simulink library "wt_blockset_v3"  (Simulink 6.0)
settings: Solver=ode45  SolverMode=SingleTasking  StartTime=0.0  StopTime=10.0  RelTol=1e-3
undefined symbols (not defined in the file): f1, get, j, Kmode, Type, u0
libraries: simulink_extras x12, simulink3 x5, simulink x4, dspinverses x1, dspmtrx3 x1, dspsnks4 x1
(part 6 of 7)

== system wt_blockset_v3/Electrical Machinery/Simulink Blocks  based Models/RMS  Squirrel Cage Induction Machine/Steady State Model ==
  Vs : Inport  Port=1  LatchInput=off
  omg : Inport  Port=2  LatchInput=off
  Complex to Magnitude-Angle : ComplexToMagnitudeAngle
  Mux : Mux
  Mux1 : Mux  Inputs=2
  Product : Product  Inputs=*/  SaturateOnIntegerOverflow=on  InputSameDT=on
  Real-Imag to Complex : RealImagToComplex
  Selector : Selector  Elements=[1]  InputPortWidth=4
  electromagnetique torque : Fcn  Expr=3*p*Xm^2*u(1)^2*u(2)*u(3)/((Rs*u(3)+(Xm^2-Xs*u(4))*u(2))^2+(u(3)*Xs+u(2)*Rs*u(4))^2)/omg_base
  equivalent reactance : Fcn  Expr=(((u(3)/u(2))^2)*Xs-u(4)*(Xm^2-Xs*u(4)))/((u(3)/u(2))^2+u(4)^2)
  equivalent resistance : Fcn  Expr=(Rs*(u(3)/u(2))^2+Xm^2*u(3)/u(2)+Rs*u(4))/((u(3)/u(2))^2+u(4)^2)
  m<->g : Fcn  Expr=u(1)*(u(2) >=0)-(pi-u(1))*(u(2) < 0)
  rad->deg : Gain  Gain=180/pi  SaturateOnIntegerOverflow=on
  rotor reactance : Fcn  Expr=Xsgm_r*(abs(u(1))<=sbd)+(Xsgm_r*((kx-1)*abs(u(1))+(1-kx*sbd))/(1-sbd))*(abs(u(1))>sbd)+Xm
  rotor resistance : Fcn  Expr=Rr*(abs(u(1))<=sbd)+(Rr*((kr-1)*abs(u(1))+(1-kr*sbd))/(1-sbd))*(abs(u(1))>sbd)
  slip : Fcn  Expr=1-u(1)/omg_base
  Te : Outport
  Iph : Outport  Port=2
  phase_angle : Outport  Port=3
  wires:
  m<->g/1 -> rad->deg/1
  Mux1/1 -> m<->g/1
  Complex to Magnitude-Angle/2 -> Mux1/1
  Real-Imag to Complex/1 -> Complex to Magnitude-Angle/1
  Product/1 -> Iph/1
  Selector/1 -> Product/1
  Complex to Magnitude-Angle/1 -> Product/2
  rad->deg/1 -> phase_angle/1
  equivalent reactance/1 -> Real-Imag to Complex/2
  equivalent resistance/1 -> Real-Imag to Complex/1
  Mux/1 -> equivalent reactance/1, Selector/1, electromagnetique torque/1, equivalent resistance/1
  rotor reactance/1 -> Mux/4
  electromagnetique torque/1 -> Te/1
  rotor resistance/1 -> Mux/3
  slip/1 -> Mux1/2, rotor reactance/1, rotor resistance/1, Mux/2
  Vs/1 -> Mux/1
  omg/1 -> slip/1

== system wt_blockset_v3/Electrical Machinery/Simulink Blocks  based Models/Salient-Pole Synchronous Machine constant parameters/Mathematical model ==
  usdq : Inport  Port=1  LatchInput=off
  uf : Inport  Port=2  LatchInput=off
  omgr : Inport  Port=3  LatchInput=off
  Demux : Demux  Outputs=2
  Integrator{1..5} (5 alike) : Integrator
  Mux : Mux  Inputs=9
  Mux1 : Mux  Inputs=3
  Telm : Fcn  Expr=1.5*p*((Lmd-Lmq)*u[1]*u[2]+Lmq*u[2]*(u[3]+u[4])-Lmq*u[5]*u[1])
  dif/dt : Fcn  Expr=a31*u[1]+a32*u[9]*u[2]+a33*u[3]+a34*u[4]+a35*u[9]*u[5]+a36*u[6]+a37*u[8]
  dird/dt : Fcn  Expr=a41*u[1]+a42*u[9]*u[2]+a43*u[3]+a44*u[4]+a45*u[9]*u[5]+a46*u[6]+a47*u[8]
  dirq/dt : Fcn  Expr=a51*u[9]*u[1]+a52*u[2]+a53*u[9]*u[3]+a54*u[9]*u[4]+a55*u[5]+a56*u[7]
  disd/dt : Fcn  Expr=a11*u[1]+a12*u[9]*u[2]+a13*u[3]+a14*u[4]+a15*u[9]*u[5]+a16*u[6]+a17*u[8]
  disq/dt : Fcn  Expr=a21*u[9]*u[1]+a22*u[2]+a23*u[9]*u[3]+a24*u[9]*u[4]+a25*u[5]+a26*u[7]
  dq / abc : Subsystem
  isd : Selector  Elements=[1]  InputPortWidth=9
  isq : Selector  Elements=[2]  InputPortWidth=9
  Te : Outport  InitialOutput=0
  is_UVW : Outport  Port=2  InitialOutput=0
  wires:
  Mux/1 -> disd/dt/1, disq/dt/1, dif/dt/1, dird/dt/1, dirq/dt/1, Telm/1, isd/1, isq/1
  omgr/1 -> Mux/9
  uf/1 -> Mux/8
  disd/dt/1 -> Integrator4/1
  disq/dt/1 -> Integrator1/1
  dif/dt/1 -> Integrator2/1
  dird/dt/1 -> Integrator3/1
  dirq/dt/1 -> Integrator5/1
  Integrator5/1 -> Mux/5
  Integrator3/1 -> Mux/4
  Integrator2/1 -> Mux/3
  Integrator1/1 -> Mux/2
  Integrator4/1 -> Mux/1
  Telm/1 -> Te/1
  Demux/2 -> Mux/7
  Demux/1 -> Mux/6
  usdq/1 -> Demux/1
  dq / abc/1(A) -> Mux1/1
  dq / abc/2(B) -> Mux1/2
  dq / abc/3(C) -> Mux1/3
  Mux1/1 -> is_UVW/1
  [theta] -> dq / abc/3(theta)
  isd/1 -> dq / abc/1(D)
  isq/1 -> dq / abc/2(Q)

== system wt_blockset_v3/Electrical Machinery/Simulink Blocks  based Models/Salient-Pole Synchronous Machine constant parameters/abc-dq ==
  ABC : Inport  Port=1  LatchInput=off
  theta : Inport  Port=2  LatchInput=off
  Mux : Mux  Inputs=[3 1]
  Mux1 : Mux  Inputs=2
  d : Fcn  Expr=2*(u[1]*cos(u[4])+u[2]*cos(u[4]-2*pi/3)+u[3]*cos(u[4]+2*pi/3))/3
  q : Fcn  Expr=-2*(u[1]*sin(u[4])+u[2]*sin(u[4]-2*pi/3)+u[3]*sin(u[4]+2*pi/3))/3
  DQ : Outport  InitialOutput=0
  wires:
  Mux/1 -> d/1, q/1
  ABC/1 -> Mux/1
  Mux1/1 -> DQ/1
  d/1 -> Mux1/1
  q/1 -> Mux1/2
  theta/1 -> Mux/2

== system wt_blockset_v3/Electrical Machinery/Simulink Blocks  based Models/Squirrel Cage Induction Machine constant parameters/Derivatives ==
  vdqs : Inport  Port=1  LatchInput=off
  omega : Inport  Port=2  LatchInput=off
  Mux : Mux  Inputs=[1 1 1 1 2 1]
  Selector : Selector  Elements=[7]  InputPortWidth=7
  Selector1 : Selector  Elements=[1 2]  InputPortWidth=7
  didr/dt : Fcn  Expr=((Rs*Lm*u(1))/(Lss*Lsr)-Lm*u(7)*u(2)/Lsr-Rr*u(3)/Lsr-(Lm^2*u(7)*u(4))/(Lss*Lsr)-(Lm*u(5))/(Lss*Lsr))/sigma
  dids/dt : Fcn  Expr=(-Rs*u(1)/Lss+u(7)*u(2)+(Lm*Rr*u(3))/(Lss*Lsr)+Lm*u(7)*u(4)/Lss+u(5)/Lss)/sigma
  diqr/dt : Fcn  Expr=(Lm*u(7)*u(1)/Lsr+(Rs*Lm*u(2))/(Lss*Lsr)+(Lm^2*u(7)*u(3))/(Lss*Lsr)-Rr*u(4)/Lsr-(Lm*u(6))/(Lss*Lsr))/sigma
  diqs/dt : Fcn  Expr=(-u(7)*u(1)-Rs*u(2)/Lss-Lm*u(7)*u(3)/Lss+(Rr*Lm*u(4))/(Lss*Lsr)+u(6)/Lss)/sigma
  electromagnetique torque : Fcn  Expr=1.5*Lm*p*(u(2)*u(3)-u(1)*u(4))
  int_1 : Integrator  InitialCondition=x0(1)
  int_2 : Integrator  InitialCondition=x0(2)
  int_3 : Integrator  InitialCondition=x0(3)
  int_4 : Integrator  InitialCondition=x0(4)
  int_5 : Integrator  InitialCondition=x0(5)
  idqs : Outport
  Te : Outport  Port=2
  tag scope: theta=global
  wires:
  Selector1/1 -> idqs/1
  diqs/dt/1 -> int_2/1
  Selector/1 -> int_5/1
  int_5/1 -> [theta]  "theta"
  electromagnetique torque/1 -> Te/1
  diqr/dt/1 -> int_4/1
  didr/dt/1 -> int_3/1
  dids/dt/1 -> int_1/1
  Mux/1 -> Selector1/1, Selector/1, electromagnetique torque/1, diqr/dt/1, didr/dt/1, diqs/dt/1, dids/dt/1
  omega/1 -> Mux/6  "omega_rot"
  vdqs/1 -> Mux/5  "vdqs"
  int_4/1 -> Mux/4  "iqr"
  int_3/1 -> Mux/3  "idr"
  int_2/1 -> Mux/2  "iqs"
  int_1/1 -> Mux/1  "ids"

== system wt_blockset_v3/Electrical Machinery/Simulink Blocks  based Models/Squirrel Cage Induction Machine constant parameters/abc-dq ==
  ABC : Inport  Port=1  LatchInput=off
  theta : Inport  Port=2  LatchInput=off
  Mux : Mux  Inputs=[3 1]
  Mux1 : Mux  Inputs=2
  d : Fcn  Expr=2*(u[1]*cos(u[4])+u[2]*cos(u[4]-2*pi/3)+u[3]*cos(u[4]+2*pi/3))/3
  q : Fcn  Expr=-2*(u[1]*sin(u[4])+u[2]*sin(u[4]-2*pi/3)+u[3]*sin(u[4]+2*pi/3))/3
  DQ : Outport  InitialOutput=0
  wires:
  q/1 -> Mux1/2  "vqs"
  theta/1 -> Mux/2
  Mux1/1 -> DQ/1
  d/1 -> Mux1/1  "vds"
  ABC/1 -> Mux/1
  Mux/1 -> q/1, d/1

== system wt_blockset_v3/Electrical Machinery/Simulink Blocks  based Models/Squirrel Cage Induction Machine constant parameters/dq / abc ==
  DQ : Inport  Port=1  LatchInput=off
  theta : Inport  Port=2  LatchInput=off
  Mux : Mux  Inputs=[2 1]
  Mux1 : Mux  Inputs=3
  va : Fcn  Expr=u[1]*cos(u[3])-u[2]*sin(u[3])
  vb : Fcn  Expr=u[1]*cos(u[3]-2*pi/3)-u[2]*sin(u[3]-2*pi/3)
  vc : Fcn  Expr=u[1]*cos(u[3]+2*pi/3)-u[2]*sin(u[3]+2*pi/3)
  ABC : Outport  InitialOutput=0
  wires:
  theta/1 -> Mux/2
  Mux1/1 -> ABC/1
  vc/1 -> Mux1/3
  vb/1 -> Mux1/2
  va/1 -> Mux1/1
  DQ/1 -> Mux/1
  Mux/1 -> va/1, vb/1, vc/1

== system wt_blockset_v3/Electrical Machinery/Simulink Blocks  based Models/Squirrel Cage Induction Machine constant parameters/phase ->line ==
  In : Inport  Port=1  LatchInput=off
  Mux1 : Mux  Inputs=3
  iab : Fcn  Expr=u(1)-u(2)
  ibc : Fcn  Expr=u(2)-u(3)
  ica : Fcn  Expr=u(3)-u(1)
  Out : Outport
  wires:
  iab/1 -> Mux1/1
  ibc/1 -> Mux1/2
  ica/1 -> Mux1/3
  Mux1/1 -> Out/1
  In/1 -> iab/1, ibc/1, ica/1

== system wt_blockset_v3/Electrical Machinery/Simulink Blocks  based Models/Squirrel Cage  Induction Machine  with Deep Bar Effect/Derivatives ==
  note: DQ Model Of Squirrel-Cage Induction Machine with deep bar effect
  vdqs : Inport  Port=1  LatchInput=off
  omega : Inport  Port=2  LatchInput=off
  Mux : Mux  Inputs=[1 1 1 1 2 1 1 1]
  Selector : Selector  Elements=[7]  InputPortWidth=9
  Selector1 : Selector  Elements=[1 2]  InputPortWidth=9
  didr/dt : Fcn  Expr=((Rs*Lm*u(1))/(Lss*(u(9)+Lm))-Lm*u(7)*u(2)/(u(9)+Lm)-u(8)*u(3)/(u(9)+Lm)-(Lm^2*u(7)*u(4))/(Lss*(u(9)+Lm))-(Lm*u(5))/(Lss*(u(9)+Lm)))/(1-Lm^2/(Lss*(u(9)+Lm)))
  dids/dt : Fcn  Expr=(-Rs*u(1)/Lss+u(7)*u(2)+(Lm*u(8)*u(3))/(Lss*(u(9)+Lm))+Lm*u(7)*u(4)/Lss+u(5)/Lss)/(1-Lm^2/(Lss*(u(9)+Lm)))
  diqr/dt : Fcn  Expr=(Lm*u(7)*u(1)/(u(9)+Lm)+(Rs*Lm*u(2))/(Lss*(u(9)+Lm))+(Lm^2*u(7)*u(3))/(Lss*(u(9)+Lm))-u(8)*u(4)/(u(9)+Lm)-(Lm*u(6))/(Lss*(u(9)+Lm)))/(1-Lm^2/(Lss*(u(9)+Lm)))
  diqs/dt : Fcn  Expr=(-u(7)*u(1)-Rs*u(2)/Lss-Lm*u(7)*u(3)/Lss+(u(8)*Lm*u(4))/(Lss*(u(9)+Lm))+u(6)/Lss)/(1-Lm^2/(Lss*(u(9)+Lm)))
  electromagnetic torque : Fcn  Expr=1.5*Lm*p*(u(2)*u(3)-u(1)*u(4))
  int_1 : Integrator  InitialCondition=x0(1)
  int_2 : Integrator  InitialCondition=x0(2)
  int_3 : Integrator  InitialCondition=x0(3)
  int_4 : Integrator  InitialCondition=x0(4)
  int_5 : Integrator  InitialCondition=x0(5)
  rotor reactance : Fcn  Expr=Lsgmr*(abs(u(1))<=sbd)+(Lsgmr*((kx-1)*abs(u(1))+(1-kx*sbd))/(1-sbd))*(abs(u(1))>sbd)
  rotor resistance : Fcn  Expr=Rr*(abs(u(1))<=sbd)+(Rr*((kr-1)*abs(u(1))+(1-kr*sbd))/(1-sbd))*(abs(u(1))>sbd)
  slip : Fcn  Expr=1-u(1)/omg_base
  idqs : Outport
  Te : Outport  Port=2
  tag scope: theta=global
  wires:
  rotor reactance/1 -> Mux/8
  slip/1 -> rotor reactance/1, rotor resistance/1  "omega_rot"
  rotor resistance/1 -> Mux/7
  Selector1/1 -> idqs/1
  diqs/dt/1 -> int_2/1
  Selector/1 -> int_5/1
  int_5/1 -> [theta]  "theta"
  electromagnetic torque/1 -> Te/1
  diqr/dt/1 -> int_4/1
  didr/dt/1 -> int_3/1
  dids/dt/1 -> int_1/1
  Mux/1 -> Selector1/1, Selector/1, electromagnetic torque/1, diqr/dt/1, didr/dt/1, diqs/dt/1, dids/dt/1
  omega/1 -> Mux/6, slip/1  "omega_rot"
  vdqs/1 -> Mux/5  "vdqs"
  int_4/1 -> Mux/4  "iqr"
  int_3/1 -> Mux/3  "idr"
  int_2/1 -> Mux/2  "iqs"
  int_1/1 -> Mux/1  "ids"

== system wt_blockset_v3/Electrical Machinery/Simulink Blocks  based Models/Squirrel Cage  Induction Machine  with Deep Bar Effect/Subsystem1 ==
  DQ : Inport  Port=1  LatchInput=off
  theta : Inport  Port=2  LatchInput=off
  Mux : Mux  Inputs=[2 1]
  Mux1 : Mux  Inputs=3
  va : Fcn  Expr=u[1]*cos(u[3])-u[2]*sin(u[3])
  vb : Fcn  Expr=u[1]*cos(u[3]-2*pi/3)-u[2]*sin(u[3]-2*pi/3)
  vc : Fcn  Expr=u[1]*cos(u[3]+2*pi/3)-u[2]*sin(u[3]+2*pi/3)
  ABC : Outport  InitialOutput=0
  wires:
  theta/1 -> Mux/2
  Mux1/1 -> ABC/1
  vc/1 -> Mux1/3
  vb/1 -> Mux1/2
  va/1 -> Mux1/1
  DQ/1 -> Mux/1
  Mux/1 -> va/1, vb/1, vc/1

== system wt_blockset_v3/Electrical Machinery/Simulink Blocks  based Models/Squirrel Cage  Induction Machine  with Deep Bar Effect/abc-dq ==
  ABC : Inport  Port=1  LatchInput=off
  theta : Inport  Port=2  LatchInput=off
  Mux : Mux  Inputs=[3 1]
  Mux1 : Mux  Inputs=2
  d : Fcn  Expr=2*(u[1]*cos(u[4])+u[2]*cos(u[4]-2*pi/3)+u[3]*cos(u[4]+2*pi/3))/3
  q : Fcn  Expr=-2*(u[1]*sin(u[4])+u[2]*sin(u[4]-2*pi/3)+u[3]*sin(u[4]+2*pi/3))/3
  DQ : Outport  InitialOutput=0
  wires:
  q/1 -> Mux1/2  "vqs"
  theta/1 -> Mux/2
  Mux1/1 -> DQ/1
  d/1 -> Mux1/1  "vds"
  ABC/1 -> Mux/1
  Mux/1 -> q/1, d/1

== system wt_blockset_v3/Electrical Machinery/Simulink Blocks  based Models/Squirrel Cage  Induction Machine  with Deep Bar Effect/phase ->line ==
  In : Inport  Port=1  LatchInput=off
  Mux1 : Mux  Inputs=3
  iab : Fcn  Expr=u(1)-u(2)
  ibc : Fcn  Expr=u(2)-u(3)
  ica : Fcn  Expr=u(3)-u(1)
  Out : Outport
  wires:
  In/1 -> ica/1, ibc/1, iab/1
  Mux1/1 -> Out/1
  ica/1 -> Mux1/3
  ibc/1 -> Mux1/2
  iab/1 -> Mux1/1

== system wt_blockset_v3/Electrical Machinery/Simulink Blocks  based Models/Wound Rotor Induction Machine constant parameters/Subsystem1 ==
  DQ : Inport  Port=1  LatchInput=off
  theta : Inport  Port=2  LatchInput=off
  Mux : Mux  Inputs=[2 1]
  Mux1 : Mux  Inputs=3
  va : Fcn  Expr=u[1]*cos(u[3])-u[2]*sin(u[3])
  vb : Fcn  Expr=u[1]*cos(u[3]-2*pi/3)-u[2]*sin(u[3]-2*pi/3)
  vc : Fcn  Expr=u[1]*cos(u[3]+2*pi/3)-u[2]*sin(u[3]+2*pi/3)
  ABC : Outport  InitialOutput=0
  wires:
  theta/1 -> Mux/2
  Mux1/1 -> ABC/1
  vc/1 -> Mux1/3
  vb/1 -> Mux1/2
  va/1 -> Mux1/1
  DQ/1 -> Mux/1
  Mux/1 -> va/1, vb/1, vc/1

== system wt_blockset_v3/Electrical Machinery/Simulink Blocks  based Models/Wound Rotor Induction Machine constant parameters/Subsystem2 ==
  DQ : Inport  Port=1  LatchInput=off
  theta : Inport  Port=2  LatchInput=off
  Mux : Mux  Inputs=[2 1]
  Mux1 : Mux  Inputs=3
  va : Fcn  Expr=u[1]*cos(u[3])-u[2]*sin(u[3])
  vb : Fcn  Expr=u[1]*cos(u[3]-2*pi/3)-u[2]*sin(u[3]-2*pi/3)
  vc : Fcn  Expr=u[1]*cos(u[3]+2*pi/3)-u[2]*sin(u[3]+2*pi/3)
  ABC : Outport  InitialOutput=0
  wires:
  theta/1 -> Mux/2
  Mux/1 -> vc/1, vb/1, va/1
  DQ/1 -> Mux/1
  va/1 -> Mux1/1
  vb/1 -> Mux1/2
  vc/1 -> Mux1/3
  Mux1/1 -> ABC/1

== system wt_blockset_v3/Electrical Machinery/Simulink Blocks  based Models/Wound Rotor Induction Machine constant parameters/Voltage equations ==
  vdqs : Inport  Port=1  LatchInput=off
  vdqr : Inport  Port=2  LatchInput=off
  omega : Inport  Port=3  LatchInput=off
  Mux : Mux  Inputs=[1 1 1 1 2 2 1]
  Selector : Selector  Elements=[1 2]  InputPortWidth=9
  Selector1 : Selector  Elements=[3 4]  InputPortWidth=9
  Selector2 : Selector  Elements=[9]  InputPortWidth=9
  didr/dt : Fcn  Expr=(Rs*Lm*u(1)/(Lss*Lsr)-Lm*u(9)*u(2)/Lsr-Rr*u(3)/Lsr-((Lm^2)*u(9)*u(4))/(Lss*Lsr)-Lm*u(5)/(Lss*Lsr)+u(7)/Lsr)/sigma
  dids/dt : Fcn  Expr=(-Rs*u(1)/Lss+u(9)*u(2)+(Lm*Rr*u(3))/(Lss*Lsr)+Lm*u(9)*u(4)/Lss+u(5)/Lss-Lm*u(7)/(Lss*Lsr))/sigma
  diqr/dt : Fcn  Expr=(Lm*u(9)*u(1)/Lsr+Rs*Lm*u(2)/(Lss*Lsr)+((Lm^2)*u(9)*u(3))/(Lss*Lsr)-Rr*u(4)/Lsr-Lm*u(6)/(Lss*Lsr)+u(8)/Lsr)/sigma
  diqs/dt : Fcn  Expr=(-u(9)*u(1)-Rs*u(2)/Lss-Lm*u(9)*u(3)/Lss+(Rr*Lm*u(4))/(Lss*Lsr)+u(6)/Lss-Lm*u(8)/(Lss*Lsr))/sigma
  electromagnetique torque : Fcn  Expr=1.5*Lm*p*(u(2)*u(3)-u(1)*u(4))
  int_1 : Integrator  InitialCondition=x0(1)
  int_2 : Integrator  InitialCondition=x0(2)
  int_3 : Integrator  InitialCondition=x0(3)
  int_4 : Integrator  InitialCondition=x0(4)
  int_5 : Integrator  InitialCondition=x0(5)
  idqs : Outport
  idqr : Outport  Port=2
  Te : Outport  Port=3
  tag scope: theta=global
  wires:
  Selector1/1 -> idqr/1
  Selector/1 -> idqs/1
  vdqr/1 -> Mux/6
  omega/1 -> Mux/7  "omega_rot"
  Selector2/1 -> int_5/1
  int_5/1 -> [theta]  "theta"
  electromagnetique torque/1 -> Te/1
  diqr/dt/1 -> int_4/1  "diqr"
  didr/dt/1 -> int_3/1  "didr"
  diqs/dt/1 -> int_2/1  "diqs"
  dids/dt/1 -> int_1/1  "dids"
  Mux/1 -> Selector1/1, Selector/1, Selector2/1, electromagnetique torque/1, diqr/dt/1, didr/dt/1, diqs/dt/1, dids/dt/1
  vdqs/1 -> Mux/5
  int_4/1 -> Mux/4  "iqr"
  int_3/1 -> Mux/3  "idr"
  int_2/1 -> Mux/2  "iqs"
  int_1/1 -> Mux/1  "ids"

== system wt_blockset_v3/Electrical Machinery/Simulink Blocks  based Models/Wound Rotor Induction Machine constant parameters/abc-dq ==
  ABC : Inport  Port=1  LatchInput=off
  theta : Inport  Port=2  LatchInput=off
  Mux : Mux  Inputs=[3 1]
  Mux1 : Mux  Inputs=2
  d : Fcn  Expr=2*(u[1]*cos(u[4])+u[2]*cos(u[4]-2*pi/3)+u[3]*cos(u[4]+2*pi/3))/3
  q : Fcn  Expr=-2*(u[1]*sin(u[4])+u[2]*sin(u[4]-2*pi/3)+u[3]*sin(u[4]+2*pi/3))/3
  DQ : Outport  InitialOutput=0
  wires:
  q/1 -> Mux1/2  "vqs"
  theta/1 -> Mux/2
  Mux1/1 -> DQ/1
  d/1 -> Mux1/1  "vds"
  ABC/1 -> Mux/1
  Mux/1 -> q/1, d/1

== system wt_blockset_v3/Electrical Machinery/Simulink Blocks  based Models/Wound Rotor Induction Machine constant parameters/abc-dq1 ==
  ABC : Inport  Port=1  LatchInput=off
  theta : Inport  Port=2  LatchInput=off
  Mux : Mux  Inputs=[3 1]
  Mux1 : Mux  Inputs=2
  d : Fcn  Expr=2*(u[1]*cos(u[4])+u[2]*cos(u[4]-2*pi/3)+u[3]*cos(u[4]+2*pi/3))/3
  q : Fcn  Expr=-2*(u[1]*sin(u[4])+u[2]*sin(u[4]-2*pi/3)+u[3]*sin(u[4]+2*pi/3))/3
  DQ : Outport  InitialOutput=0
  wires:
  theta/1 -> Mux/2
  Mux/1 -> d/1, q/1
  ABC/1 -> Mux/1
  d/1 -> Mux1/1  "vdr"
  q/1 -> Mux1/2  "vqr"
  Mux1/1 -> DQ/1

== system wt_blockset_v3/Electrical Machinery/Simulink Blocks  based Models/Wound Rotor Induction Machine with Deep Bar Effect /Subsystem1 ==
  DQ : Inport  Port=1  LatchInput=off
  theta : Inport  Port=2  LatchInput=off
  Mux : Mux  Inputs=[2 1]
  Mux1 : Mux  Inputs=3
  va : Fcn  Expr=u[1]*cos(u[3])-u[2]*sin(u[3])
  vb : Fcn  Expr=u[1]*cos(u[3]-2*pi/3)-u[2]*sin(u[3]-2*pi/3)
  vc : Fcn  Expr=u[1]*cos(u[3]+2*pi/3)-u[2]*sin(u[3]+2*pi/3)
  ABC : Outport  InitialOutput=0
  wires:
  Mux/1 -> vc/1, vb/1, va/1
  DQ/1 -> Mux/1
  va/1 -> Mux1/1
  vb/1 -> Mux1/2
  vc/1 -> Mux1/3
  Mux1/1 -> ABC/1
  theta/1 -> Mux/2

== system wt_blockset_v3/Electrical Machinery/Simulink Blocks  based Models/Wound Rotor Induction Machine with Deep Bar Effect /Subsystem2 ==
  DQ : Inport  Port=1  LatchInput=off
  theta : Inport  Port=2  LatchInput=off
  Mux : Mux  Inputs=[2 1]
  Mux1 : Mux  Inputs=3
  va : Fcn  Expr=u[1]*cos(u[3])-u[2]*sin(u[3])
  vb : Fcn  Expr=u[1]*cos(u[3]-2*pi/3)-u[2]*sin(u[3]-2*pi/3)
  vc : Fcn  Expr=u[1]*cos(u[3]+2*pi/3)-u[2]*sin(u[3]+2*pi/3)
  ABC : Outport  InitialOutput=0
  wires:
  Mux1/1 -> ABC/1
  vc/1 -> Mux1/3
  vb/1 -> Mux1/2
  va/1 -> Mux1/1
  DQ/1 -> Mux/1
  Mux/1 -> va/1, vb/1, vc/1
  theta/1 -> Mux/2

== system wt_blockset_v3/Electrical Machinery/Simulink Blocks  based Models/Wound Rotor Induction Machine with Deep Bar Effect /Voltage equations ==
  vdqs : Inport  Port=1  LatchInput=off
  vdqr : Inport  Port=2  LatchInput=off
  omega : Inport  Port=3  LatchInput=off
  Mux : Mux  Inputs=[1 1 1 1 2 2 1 1 1]
  Selector : Selector  Elements=[1 2]  InputPortWidth=11
  Selector1 : Selector  Elements=[3 4]  InputPortWidth=11
  Selector2 : Selector  Elements=[9]  InputPortWidth=11
  didr/dt : Fcn  Expr=(Rs*Lm*u(1)/(Lss*u(11))-Lm*u(9)*u(2)/u(11)-u(10)*u(3)/u(11)-((Lm^2)*u(9)*u(4))/(Lss*u(11))-Lm*u(5)/(Lss*u(11))+u(7)/u(11))/(1-(Lm*Lm)/(Lss*u(11)))
  dids/dt : Fcn  Expr=(-Rs*u(1)/Lss+u(9)*u(2)+(Lm*u(10)*u(3))/(Lss*u(11))+Lm*u(9)*u(4)/Lss+u(5)/Lss-Lm*u(7)/(Lss*u(11)))/(1-(Lm*Lm)/(Lss*u(11)))
  diqr/dt : Fcn  Expr=(Lm*u(9)*u(1)/u(11)+Rs*Lm*u(2)/(Lss*u(11))+((Lm^2)*u(9)*u(3))/(Lss*u(11))-u(10)*u(4)/u(11)-Lm*u(6)/(Lss*u(11))+u(8)/u(11))/(1-(Lm*Lm)/(Lss*u(11)))
  diqs/dt : Fcn  Expr=(-u(9)*u(1)-Rs*u(2)/Lss-Lm*u(9)*u(3)/Lss+(u(10)*Lm*u(4))/(Lss*u(11))+u(6)/Lss-Lm*u(8)/(Lss*u(11)))/(1-(Lm*Lm)/(Lss*u(11)))
  electromagnetique torque : Fcn  Expr=1.5*Lm*p*(u(2)*u(3)-u(1)*u(4))
  int_1 : Integrator  InitialCondition=x0(1)
  int_2 : Integrator  InitialCondition=x0(2)
  int_3 : Integrator  InitialCondition=x0(3)
  int_4 : Integrator  InitialCondition=x0(4)
  int_5 : Integrator  InitialCondition=x0(5)
  rotor reactance : Fcn  Expr=Lsgmr*(abs(u(1))<=sbd)+(Lsgmr*((kx-1)*abs(u(1))+(1-kx*sbd))/(1-sbd))*(abs(u(1))>sbd)+Lm
  rotor resistance : Fcn  Expr=Rr*(abs(u(1))<=sbd)+(Rr*((kr-1)*abs(u(1))+(1-kr*sbd))/(1-sbd))*(abs(u(1))>sbd)
  slip : Fcn  Expr=1-u(1)/omg_base
  idqs : Outport
  idqr : Outport  Port=2
  Te : Outport  Port=3
  tag scope: theta=global
  wires:
  int_1/1 -> Mux/1  "ids"
  int_2/1 -> Mux/2  "iqs"
  int_3/1 -> Mux/3  "idr"
  int_4/1 -> Mux/4  "iqr"
  vdqs/1 -> Mux/5
  dids/dt/1 -> int_1/1  "dids"
  diqs/dt/1 -> int_2/1  "diqs"
  didr/dt/1 -> int_3/1  "didr"
  diqr/dt/1 -> int_4/1  "diqr"
  electromagnetique torque/1 -> Te/1
  int_5/1 -> [theta]  "theta"
  Selector2/1 -> int_5/1
  omega/1 -> Mux/7, slip/1  "omega_rot"
  vdqr/1 -> Mux/6
  Selector/1 -> idqs/1
  Selector1/1 -> idqr/1
  slip/1 -> rotor resistance/1, rotor reactance/1
  rotor resistance/1 -> Mux/8
  rotor reactance/1 -> Mux/9
  Mux/1 -> diqr/dt/1, didr/dt/1, diqs/dt/1, dids/dt/1, electromagnetique torque/1, Selector2/1, Selector/1, Selector1/1

== system wt_blockset_v3/Electrical Machinery/Simulink Blocks  based Models/Wound Rotor Induction Machine with Deep Bar Effect /abc-dq ==
  ABC : Inport  Port=1  LatchInput=off
  theta : Inport  Port=2  LatchInput=off
  Mux : Mux  Inputs=[3 1]
  Mux1 : Mux  Inputs=2
  d : Fcn  Expr=2*(u[1]*cos(u[4])+u[2]*cos(u[4]-2*pi/3)+u[3]*cos(u[4]+2*pi/3))/3
  q : Fcn  Expr=-2*(u[1]*sin(u[4])+u[2]*sin(u[4]-2*pi/3)+u[3]*sin(u[4]+2*pi/3))/3
  DQ : Outport  InitialOutput=0
  wires:
  Mux/1 -> d/1, q/1
  ABC/1 -> Mux/1
  d/1 -> Mux1/1  "vds"
  Mux1/1 -> DQ/1
  theta/1 -> Mux/2
  q/1 -> Mux1/2  "vqs"

== system wt_blockset_v3/Electrical Machinery/Simulink Blocks  based Models/Wound Rotor Induction Machine with Deep Bar Effect /abc-dq1 ==
  ABC : Inport  Port=1  LatchInput=off
  theta : Inport  Port=2  LatchInput=off
  Mux : Mux  Inputs=[3 1]
  Mux1 : Mux  Inputs=2
  d : Fcn  Expr=2*(u[1]*cos(u[4])+u[2]*cos(u[4]-2*pi/3)+u[3]*cos(u[4]+2*pi/3))/3
  q : Fcn  Expr=-2*(u[1]*sin(u[4])+u[2]*sin(u[4]-2*pi/3)+u[3]*sin(u[4]+2*pi/3))/3
  DQ : Outport  InitialOutput=0
  wires:
  Mux1/1 -> DQ/1
  q/1 -> Mux1/2  "vqr"
  d/1 -> Mux1/1  "vdr"
  ABC/1 -> Mux/1
  Mux/1 -> q/1, d/1
  theta/1 -> Mux/2

== system wt_blockset_v3/Grid Models/Circuit breaker/Circuit breaker1/delay tc ==
  note: AND  used to suppress
      | spurious operation when
      | input goes from high to low
  in_1 : Inport  Port=1  LatchInput=off
  Logical Operator : Logic  Operator=XOR
  Logical Operator1 : Logic
  Transport Delay1 : TransportDelay  DelayTime=tc  BufferSize=20000
  out_1 : Outport
  wires:
  Transport Delay1/1 -> Logical Operator/2
  in_1/1 -> Logical Operator/1, Transport Delay1/1, Logical Operator1/1
  Logical Operator1/1 -> out_1/1
  Logical Operator/1 -> Logical Operator1/2

== system wt_blockset_v3/Grid Models/Circuit breaker/Circuit breaker2/delay tc ==
  note: AND  used to suppress
      | spurious operation when
      | input goes from high to low
  in_1 : Inport  Port=1  LatchInput=off
  Logical Operator : Logic  Operator=XOR
  Logical Operator1 : Logic
  Transport Delay1 : TransportDelay  DelayTime=tc  BufferSize=20000
  out_1 : Outport
  wires:
  Logical Operator/1 -> Logical Operator1/2
  Logical Operator1/1 -> out_1/1
  in_1/1 -> Logical Operator1/1, Transport Delay1/1, Logical Operator/1
  Transport Delay1/1 -> Logical Operator/2

== system wt_blockset_v3/Grid Models/Circuit breaker/Circuit breaker3/delay tc ==
  note: AND  used to suppress
      | spurious operation when
      | input goes from high to low
  in_1 : Inport  Port=1  LatchInput=off
  Logical Operator : Logic  Operator=XOR
  Logical Operator1 : Logic
  Transport Delay1 : TransportDelay  DelayTime=tc  BufferSize=20000
  out_1 : Outport
  wires:
  Transport Delay1/1 -> Logical Operator/2
  in_1/1 -> Logical Operator/1, Transport Delay1/1, Logical Operator1/1
  Logical Operator1/1 -> out_1/1
  Logical Operator/1 -> Logical Operator1/2

== system wt_blockset_v3/Mechanical Components/Wind Model SB-2/3rd_Harmonic_Filter1/3rd harmonic Filter ==
  avg_wind : Inport  Port=1  LatchInput=off
  In : Inport  Port=2  LatchInput=off
  Coefficients : Subsystem
  Integrator : Integrator  Orientation=up
  Integrator1 : Integrator  Orientation=up
  Product : Product  SaturateOnIntegerOverflow=on
  Product1 : Product  SaturateOnIntegerOverflow=on
  Product2 : Product  Orientation=left  SaturateOnIntegerOverflow=on
  Product3 : Product  Orientation=left  SaturateOnIntegerOverflow=on
  Sum1 : Sum  Orientation=up  Inputs=++-  SaturateOnIntegerOverflow=on
  Sum2 : Sum  Orientation=up  Inputs=+|-  SaturateOnIntegerOverflow=on
  Out : Outport
  wires:
  Integrator/1 -> Product2/1, Product3/1, Out/1
  Sum1/1 -> Integrator/1
  Product/1 -> Sum1/1
  Integrator1/1 -> Sum1/2
  Product2/1 -> Sum1/3
  Sum2/1 -> Integrator1/1
  Product3/1 -> Sum2/2
  Product1/1 -> Sum2/1
  In/1 -> Product/1, Product1/1
  [BD] -> Product/2
  [CD] -> Product1/2
  [ED] -> Product2/2
  [FD] -> Product3/2
  Coefficients/1(BD) -> [BD]
  Coefficients/2(CD) -> [CD]
  Coefficients/3(ED) -> [ED]
  Coefficients/4(FD) -> [FD]
  avg_wind/1 -> Coefficients/1(avg_wind)

== system wt_blockset_v3/Mechanical Components/Wind Model SB-2/3rd_Harmonic_Filter2/3rd harmonic Filter ==
  avg_wind : Inport  Port=1  LatchInput=off
  In : Inport  Port=2  LatchInput=off
  Coefficients : Subsystem
  Integrator : Integrator  Orientation=up
  Integrator1 : Integrator  Orientation=up
  Product : Product  SaturateOnIntegerOverflow=on
  Product1 : Product  SaturateOnIntegerOverflow=on
  Product2 : Product  Orientation=left  SaturateOnIntegerOverflow=on
  Product3 : Product  Orientation=left  SaturateOnIntegerOverflow=on
  Sum1 : Sum  Orientation=up  Inputs=++-  SaturateOnIntegerOverflow=on
  Sum2 : Sum  Orientation=up  Inputs=+|-  SaturateOnIntegerOverflow=on
  Out : Outport
  wires:
  avg_wind/1 -> Coefficients/1(avg_wind)
  Coefficients/4(FD) -> [FD]
  Coefficients/3(ED) -> [ED]
  Coefficients/2(CD) -> [CD]
  Coefficients/1(BD) -> [BD]
  [FD] -> Product3/2
  [ED] -> Product2/2
  [CD] -> Product1/2
  [BD] -> Product/2
  In/1 -> Product1/1, Product/1
  Product1/1 -> Sum2/1
  Product3/1 -> Sum2/2
  Sum2/1 -> Integrator1/1
  Product2/1 -> Sum1/3
  Integrator1/1 -> Sum1/2
  Product/1 -> Sum1/1
  Sum1/1 -> Integrator/1
  Integrator/1 -> Out/1, Product3/1, Product2/1

== system wt_blockset_v3/Mechanical Components/Wind Model SB-2/Kaimal_Filter_1/Kaimal Filter ==
  avg_wind : Inport  Port=1  LatchInput=off
  In : Inport  Port=2  LatchInput=off
  A/D : Gain  Gain=0.0182/1.3463  SaturateOnIntegerOverflow=on
  Coefficients : Subsystem
  Integrator : Integrator  Orientation=up
  Integrator1 : Integrator  Orientation=up
  Product : Product  SaturateOnIntegerOverflow=on
  Product1 : Product  SaturateOnIntegerOverflow=on
  Product2 : Product  Orientation=left  SaturateOnIntegerOverflow=on
  Product3 : Product  Orientation=left  SaturateOnIntegerOverflow=on
  Sum : Sum  Inputs=|++  SaturateOnIntegerOverflow=on
  Sum1 : Sum  Orientation=up  Inputs=++-  SaturateOnIntegerOverflow=on
  Sum2 : Sum  Orientation=up  Inputs=+|-  SaturateOnIntegerOverflow=on
  Out : Outport
  wires:
  A/D/1 -> Sum/1
  Integrator/1 -> Sum/2
  Sum1/1 -> Integrator/1
  Product/1 -> Sum1/1
  Integrator1/1 -> Sum1/2
  Product2/1 -> Sum1/3
  Sum2/1 -> Integrator1/1
  Product3/1 -> Sum2/2
  Product1/1 -> Sum2/1
  Sum/1 -> Product2/1, Product3/1, Out/1
  In/1 -> A/D/1, Product/1, Product1/1
  [BD] -> Product/2
  [CD] -> Product1/2
  [ED] -> Product2/2
  [FD] -> Product3/2
  Coefficients/1(BD) -> [BD]
  Coefficients/2(CD) -> [CD]
  Coefficients/3(ED) -> [ED]
  Coefficients/4(FD) -> [FD]
  avg_wind/1 -> Coefficients/1(avg_wind)

== system wt_blockset_v3/Mechanical Components/Wind Model SB-2/Kaimal_Filter_2/Kaimal Filter ==
  avg_wind : Inport  Port=1  LatchInput=off
  In : Inport  Port=2  LatchInput=off
  A/D : Gain  Gain=0.0182/1.3463  SaturateOnIntegerOverflow=on
  Coefficients : Subsystem
  Integrator : Integrator  Orientation=up
  Integrator1 : Integrator  Orientation=up
  Product : Product  SaturateOnIntegerOverflow=on
  Product1 : Product  SaturateOnIntegerOverflow=on
  Product2 : Product  Orientation=left  SaturateOnIntegerOverflow=on
  Product3 : Product  Orientation=left  SaturateOnIntegerOverflow=on
  Sum : Sum  Inputs=|++  SaturateOnIntegerOverflow=on
  Sum1 : Sum  Orientation=up  Inputs=++-  SaturateOnIntegerOverflow=on
  Sum2 : Sum  Orientation=up  Inputs=+|-  SaturateOnIntegerOverflow=on
  Out : Outport
  wires:
  avg_wind/1 -> Coefficients/1(avg_wind)
  Coefficients/4(FD) -> [FD]
  Coefficients/3(ED) -> [ED]
  Coefficients/2(CD) -> [CD]
  Coefficients/1(BD) -> [BD]
  [FD] -> Product3/2
  [ED] -> Product2/2
  [CD] -> Product1/2
  [BD] -> Product/2
  In/1 -> Product1/1, Product/1, A/D/1
  Sum/1 -> Out/1, Product3/1, Product2/1
  Product1/1 -> Sum2/1
  Product3/1 -> Sum2/2
  Sum2/1 -> Integrator1/1
  Product2/1 -> Sum1/3
  Integrator1/1 -> Sum1/2
  Product/1 -> Sum1/1
  Sum1/1 -> Integrator/1
  Integrator/1 -> Sum/2
  A/D/1 -> Sum/1

== system wt_blockset_v3/Mechanical Components/Wind Model SB-2/Kaimal_Filter_3/Kaimal Filter ==
  avg_wind : Inport  Port=1  LatchInput=off
  In : Inport  Port=2  LatchInput=off
  A/D : Gain  Gain=0.0182/1.3463  SaturateOnIntegerOverflow=on
  Coefficients : Subsystem
  Integrator : Integrator  Orientation=up
  Integrator1 : Integrator  Orientation=up
  Product : Product  SaturateOnIntegerOverflow=on
  Product1 : Product  SaturateOnIntegerOverflow=on
  Product2 : Product  Orientation=left  SaturateOnIntegerOverflow=on
  Product3 : Product  Orientation=left  SaturateOnIntegerOverflow=on
  Sum : Sum  Inputs=|++  SaturateOnIntegerOverflow=on
  Sum1 : Sum  Orientation=up  Inputs=++-  SaturateOnIntegerOverflow=on
  Sum2 : Sum  Orientation=up  Inputs=+|-  SaturateOnIntegerOverflow=on
  Out : Outport
  wires:
  A/D/1 -> Sum/1
  Integrator/1 -> Sum/2
  Sum1/1 -> Integrator/1
  Product/1 -> Sum1/1
  Integrator1/1 -> Sum1/2
  Product2/1 -> Sum1/3
  Sum2/1 -> Integrator1/1
  Product3/1 -> Sum2/2
  Product1/1 -> Sum2/1
  Sum/1 -> Product2/1, Product3/1, Out/1
  In/1 -> A/D/1, Product/1, Product1/1
  [BD] -> Product/2
  [CD] -> Product1/2
  [ED] -> Product2/2
  [FD] -> Product3/2
  Coefficients/1(BD) -> [BD]
  Coefficients/2(CD) -> [CD]
  Coefficients/3(ED) -> [ED]
  Coefficients/4(FD) -> [FD]
  avg_wind/1 -> Coefficients/1(avg_wind)

== system wt_blockset_v3/Mechanical Components/Wind Model SB-2/ZERO_Harmonic_Filter/ZERO harmonic Filter ==
  avg_wind : Inport  Port=1  LatchInput=off
  In : Inport  Port=2  LatchInput=off
  Coefficients : Subsystem
  Integrator : Integrator  Orientation=up
  Integrator1 : Integrator  Orientation=up
  Product : Product  SaturateOnIntegerOverflow=on
  Product1 : Product  SaturateOnIntegerOverflow=on
  Product2 : Product  Orientation=left  SaturateOnIntegerOverflow=on
  Product3 : Product  Orientation=left  SaturateOnIntegerOverflow=on
  Sum1 : Sum  Orientation=up  Inputs=++-  SaturateOnIntegerOverflow=on
  Sum2 : Sum  Orientation=up  Inputs=+|-  SaturateOnIntegerOverflow=on
  Out : Outport
  wires:
  avg_wind/1 -> Coefficients/1(avg_wind)
  Coefficients/4(FD) -> [FD]
  Coefficients/3(ED) -> [ED]
  Coefficients/2(CD) -> [CD]
  Coefficients/1(BD) -> [BD]
  [FD] -> Product3/2
  [ED] -> Product2/2
  [CD] -> Product1/2
  [BD] -> Product/2
  In/1 -> Product1/1, Product/1
  Product1/1 -> Sum2/1
  Product3/1 -> Sum2/2
  Sum2/1 -> Integrator1/1
  Product2/1 -> Sum1/3
  Integrator1/1 -> Sum1/2
  Product/1 -> Sum1/1
  Sum1/1 -> Integrator/1
  Integrator/1 -> Out/1, Product3/1, Product2/1

== system wt_blockset_v3/Mechanical Components/Wind Model ZA-2/3rd_Harmonic_Filter1/3rd harmonic Filter ==
  avg_wind : Inport  Port=1  LatchInput=off
  In : Inport  Port=2  LatchInput=off
  Coefficients : Subsystem
  Integrator : Integrator  Orientation=up
  Integrator1 : Integrator  Orientation=up
  Product : Product  SaturateOnIntegerOverflow=on
  Product1 : Product  SaturateOnIntegerOverflow=on
  Product2 : Product  Orientation=left  SaturateOnIntegerOverflow=on
  Product3 : Product  Orientation=left  SaturateOnIntegerOverflow=on
  Sum1 : Sum  Orientation=up  Inputs=++-  SaturateOnIntegerOverflow=on
  Sum2 : Sum  Orientation=up  Inputs=+|-  SaturateOnIntegerOverflow=on
  Out : Outport
  wires:
  Integrator/1 -> Product2/1, Product3/1, Out/1
  Sum1/1 -> Integrator/1
  Product/1 -> Sum1/1
  Integrator1/1 -> Sum1/2
  Product2/1 -> Sum1/3
  Sum2/1 -> Integrator1/1
  Product3/1 -> Sum2/2
  Product1/1 -> Sum2/1
  In/1 -> Product/1, Product1/1
  [BD] -> Product/2
  [CD] -> Product1/2
  [ED] -> Product2/2
  [FD] -> Product3/2
  Coefficients/1(BD) -> [BD]
  Coefficients/2(CD) -> [CD]
  Coefficients/3(ED) -> [ED]
  Coefficients/4(FD) -> [FD]
  avg_wind/1 -> Coefficients/1(avg_wind)

== system wt_blockset_v3/Mechanical Components/Wind Model ZA-2/3rd_Harmonic_Filter2/3rd harmonic Filter ==
  avg_wind : Inport  Port=1  LatchInput=off
  In : Inport  Port=2  LatchInput=off
  Coefficients : Subsystem
  Integrator : Integrator  Orientation=up
  Integrator1 : Integrator  Orientation=up
  Product : Product  SaturateOnIntegerOverflow=on
  Product1 : Product  SaturateOnIntegerOverflow=on
  Product2 : Product  Orientation=left  SaturateOnIntegerOverflow=on
  Product3 : Product  Orientation=left  SaturateOnIntegerOverflow=on
  Sum1 : Sum  Orientation=up  Inputs=++-  SaturateOnIntegerOverflow=on
  Sum2 : Sum  Orientation=up  Inputs=+|-  SaturateOnIntegerOverflow=on
  Out : Outport
  wires:
  avg_wind/1 -> Coefficients/1(avg_wind)
  Coefficients/4(FD) -> [FD]
  Coefficients/3(ED) -> [ED]
  Coefficients/2(CD) -> [CD]
  Coefficients/1(BD) -> [BD]
  [FD] -> Product3/2
  [ED] -> Product2/2
  [CD] -> Product1/2
  [BD] -> Product/2
  In/1 -> Product1/1, Product/1
  Product1/1 -> Sum2/1
  Product3/1 -> Sum2/2
  Sum2/1 -> Integrator1/1
  Product2/1 -> Sum1/3
  Integrator1/1 -> Sum1/2
  Product/1 -> Sum1/1
  Sum1/1 -> Integrator/1
  Integrator/1 -> Out/1, Product3/1, Product2/1

== system wt_blockset_v3/Mechanical Components/Wind Model ZA-2/Kaimal_Filter_1/Kaimal Filter ==
  avg_wind : Inport  Port=1  LatchInput=off
  In : Inport  Port=2  LatchInput=off
  A/D : Gain  Gain=0.0182/1.3463  SaturateOnIntegerOverflow=on
  Coefficients : Subsystem
  Integrator : Integrator  Orientation=up
  Integrator1 : Integrator  Orientation=up
  Product : Product  SaturateOnIntegerOverflow=on
  Product1 : Product  SaturateOnIntegerOverflow=on
  Product2 : Product  Orientation=left  SaturateOnIntegerOverflow=on
  Product3 : Product  Orientation=left  SaturateOnIntegerOverflow=on
  Sum : Sum  Inputs=|++  SaturateOnIntegerOverflow=on
  Sum1 : Sum  Orientation=up  Inputs=++-  SaturateOnIntegerOverflow=on
  Sum2 : Sum  Orientation=up  Inputs=+|-  SaturateOnIntegerOverflow=on
  Out : Outport
  wires:
  A/D/1 -> Sum/1
  Integrator/1 -> Sum/2
  Sum1/1 -> Integrator/1
  Product/1 -> Sum1/1
  Integrator1/1 -> Sum1/2
  Product2/1 -> Sum1/3
  Sum2/1 -> Integrator1/1
  Product3/1 -> Sum2/2
  Product1/1 -> Sum2/1
  Sum/1 -> Product2/1, Product3/1, Out/1
  In/1 -> A/D/1, Product/1, Product1/1
  [BD] -> Product/2
  [CD] -> Product1/2
  [ED] -> Product2/2
  [FD] -> Product3/2
  Coefficients/1(BD) -> [BD]
  Coefficients/2(CD) -> [CD]
  Coefficients/3(ED) -> [ED]
  Coefficients/4(FD) -> [FD]
  avg_wind/1 -> Coefficients/1(avg_wind)

== system wt_blockset_v3/Mechanical Components/Wind Model ZA-2/Kaimal_Filter_2/Kaimal Filter ==
  avg_wind : Inport  Port=1  LatchInput=off
  In : Inport  Port=2  LatchInput=off
  A/D : Gain  Gain=0.0182/1.3463  SaturateOnIntegerOverflow=on
  Coefficients : Subsystem
  Integrator : Integrator  Orientation=up
  Integrator1 : Integrator  Orientation=up
  Product : Product  SaturateOnIntegerOverflow=on
  Product1 : Product  SaturateOnIntegerOverflow=on
  Product2 : Product  Orientation=left  SaturateOnIntegerOverflow=on
  Product3 : Product  Orientation=left  SaturateOnIntegerOverflow=on
  Sum : Sum  Inputs=|++  SaturateOnIntegerOverflow=on
  Sum1 : Sum  Orientation=up  Inputs=++-  SaturateOnIntegerOverflow=on
  Sum2 : Sum  Orientation=up  Inputs=+|-  SaturateOnIntegerOverflow=on
  Out : Outport
  wires:
  avg_wind/1 -> Coefficients/1(avg_wind)
  Coefficients/4(FD) -> [FD]
  Coefficients/3(ED) -> [ED]
  Coefficients/2(CD) -> [CD]
  Coefficients/1(BD) -> [BD]
  [FD] -> Product3/2
  [ED] -> Product2/2
  [CD] -> Product1/2
  [BD] -> Product/2
  In/1 -> Product1/1, Product/1, A/D/1
  Sum/1 -> Out/1, Product3/1, Product2/1
  Product1/1 -> Sum2/1
  Product3/1 -> Sum2/2
  Sum2/1 -> Integrator1/1
  Product2/1 -> Sum1/3
  Integrator1/1 -> Sum1/2
  Product/1 -> Sum1/1
  Sum1/1 -> Integrator/1
  Integrator/1 -> Sum/2
  A/D/1 -> Sum/1

== system wt_blockset_v3/Mechanical Components/Wind Model ZA-2/Kaimal_Filter_3/Kaimal Filter ==
  avg_wind : Inport  Port=1  LatchInput=off
  In : Inport  Port=2  LatchInput=off
  A/D : Gain  Gain=0.0182/1.3463  SaturateOnIntegerOverflow=on
  Coefficients : Subsystem
  Integrator : Integrator  Orientation=up
  Integrator1 : Integrator  Orientation=up
  Product : Product  SaturateOnIntegerOverflow=on
  Product1 : Product  SaturateOnIntegerOverflow=on
  Product2 : Product  Orientation=left  SaturateOnIntegerOverflow=on
  Product3 : Product  Orientation=left  SaturateOnIntegerOverflow=on
  Sum : Sum  Inputs=|++  SaturateOnIntegerOverflow=on
  Sum1 : Sum  Orientation=up  Inputs=++-  SaturateOnIntegerOverflow=on
  Sum2 : Sum  Orientation=up  Inputs=+|-  SaturateOnIntegerOverflow=on
  Out : Outport
  wires:
  A/D/1 -> Sum/1
  Integrator/1 -> Sum/2
  Sum1/1 -> Integrator/1
  Product/1 -> Sum1/1
  Integrator1/1 -> Sum1/2
  Product2/1 -> Sum1/3
  Sum2/1 -> Integrator1/1
  Product3/1 -> Sum2/2
  Product1/1 -> Sum2/1
  Sum/1 -> Product2/1, Product3/1, Out/1
  In/1 -> A/D/1, Product/1, Product1/1
  [BD] -> Product/2
  [CD] -> Product1/2
  [ED] -> Product2/2
  [FD] -> Product3/2
  Coefficients/1(BD) -> [BD]
  Coefficients/2(CD) -> [CD]
  Coefficients/3(ED) -> [ED]
  Coefficients/4(FD) -> [FD]
  avg_wind/1 -> Coefficients/1(avg_wind)

== system wt_blockset_v3/Mechanical Components/Wind Model ZA-2/ZERO_Harmonic_Filter/ZERO harmonic Filter ==
  avg_wind : Inport  Port=1  LatchInput=off
  In : Inport  Port=2  LatchInput=off
  Coefficients : Subsystem
  Integrator : Integrator  Orientation=up
  Integrator1 : Integrator  Orientation=up
  Product : Product  SaturateOnIntegerOverflow=on
  Product1 : Product  SaturateOnIntegerOverflow=on
  Product2 : Product  Orientation=left  SaturateOnIntegerOverflow=on
  Product3 : Product  Orientation=left  SaturateOnIntegerOverflow=on
  Sum1 : Sum  Orientation=up  Inputs=++-  SaturateOnIntegerOverflow=on
  Sum2 : Sum  Orientation=up  Inputs=+|-  SaturateOnIntegerOverflow=on
  Out : Outport
  wires:
  avg_wind/1 -> Coefficients/1(avg_wind)
  Coefficients/4(FD) -> [FD]
  Coefficients/3(ED) -> [ED]
  Coefficients/2(CD) -> [CD]
  Coefficients/1(BD) -> [BD]
  [FD] -> Product3/2
  [ED] -> Product2/2
  [CD] -> Product1/2
  [BD] -> Product/2
  In/1 -> Product1/1, Product/1
  Product1/1 -> Sum2/1
  Product3/1 -> Sum2/2
  Sum2/1 -> Integrator1/1
  Product2/1 -> Sum1/3
  Integrator1/1 -> Sum1/2
  Product/1 -> Sum1/1
  Sum1/1 -> Integrator/1
  Integrator/1 -> Out/1, Product3/1, Product2/1

== system wt_blockset_v3/Power Converters/3-phase Diode Bridge Rectifier/Diode  State Calculator/Branch A+ ==
  RST : Inport  Port=1  LatchInput=off
  Data Type Conversion : DataTypeConversion
  Demux2 : Demux  Outputs=3
  Logical Operator : Logic
  Relational Operator : RelationalOperator  InputSameDT=on
  Relational Operator1 : RelationalOperator  Operator=>  InputSameDT=on
  A : Outport  InitialOutput=0
  wires:
  Relational Operator/1 -> Logical Operator/1
  Relational Operator1/1 -> Logical Operator/2
  Logical Operator/1 -> Data Type Conversion/1
  RST/1 -> Demux2/1
  Demux2/1 -> Relational Operator/1, Relational Operator1/1
  Demux2/3 -> Relational Operator/2
  Demux2/2 -> Relational Operator1/2
  Data Type Conversion/1 -> A/1

== system wt_blockset_v3/Power Converters/3-phase Diode Bridge Rectifier/Diode  State Calculator/Branch A- ==
  RST : Inport  Port=1  LatchInput=off
  Data Type Conversion : DataTypeConversion
  Demux2 : Demux  Outputs=3
  Logical Operator : Logic
  Relational Operator : RelationalOperator  Operator=<  InputSameDT=on
  Relational Operator1 : RelationalOperator  Operator=<  InputSameDT=on
  A : Outport  InitialOutput=0
  wires:
  Demux2/2 -> Relational Operator1/2
  Demux2/3 -> Relational Operator/2
  Demux2/1 -> Relational Operator1/1, Relational Operator/1
  RST/1 -> Demux2/1
  Logical Operator/1 -> Data Type Conversion/1
  Relational Operator1/1 -> Logical Operator/2
  Relational Operator/1 -> Logical Operator/1
  Data Type Conversion/1 -> A/1

== system wt_blockset_v3/Power Converters/3-phase Diode Bridge Rectifier/Diode  State Calculator/Branch B+ ==
  RST : Inport  Port=1  LatchInput=off
  Data Type Conversion : DataTypeConversion
  Demux2 : Demux  Outputs=3
  Logical Operator : Logic
  Relational Operator : RelationalOperator  InputSameDT=on
  Relational Operator1 : RelationalOperator  Operator=>  InputSameDT=on
  B : Outport  InitialOutput=0
  wires:
  RST/1 -> Demux2/1
  Logical Operator/1 -> Data Type Conversion/1
  Relational Operator1/1 -> Logical Operator/2
  Relational Operator/1 -> Logical Operator/1
  Demux2/2 -> Relational Operator/1, Relational Operator1/1
  Demux2/1 -> Relational Operator/2
  Demux2/3 -> Relational Operator1/2
  Data Type Conversion/1 -> B/1

== system wt_blockset_v3/Power Converters/3-phase Diode Bridge Rectifier/Diode  State Calculator/Branch B- ==
  RST : Inport  Port=1  LatchInput=off
  Data Type Conversion : DataTypeConversion
  Demux2 : Demux  Outputs=3
  Logical Operator : Logic
  Relational Operator : RelationalOperator  Operator=<  InputSameDT=on
  Relational Operator1 : RelationalOperator  Operator=<  InputSameDT=on
  B : Outport  InitialOutput=0
  wires:
  Demux2/3 -> Relational Operator1/2
  Demux2/1 -> Relational Operator/2
  Demux2/2 -> Relational Operator1/1, Relational Operator/1
  Relational Operator/1 -> Logical Operator/1
  Relational Operator1/1 -> Logical Operator/2
  Logical Operator/1 -> Data Type Conversion/1
  RST/1 -> Demux2/1
  Data Type Conversion/1 -> B/1

== system wt_blockset_v3/Power Converters/3-phase Diode Bridge Rectifier/Diode  State Calculator/Branch C+ ==
  RST : Inport  Port=1  LatchInput=off
  Data Type Conversion : DataTypeConversion
  Demux2 : Demux  Outputs=3
  Logical Operator : Logic
  Relational Operator : RelationalOperator  InputSameDT=on
  Relational Operator1 : RelationalOperator  Operator=>  InputSameDT=on
  C : Outport  InitialOutput=0
  wires:
  Relational Operator/1 -> Logical Operator/1
  Relational Operator1/1 -> Logical Operator/2
  Logical Operator/1 -> Data Type Conversion/1
  RST/1 -> Demux2/1
  Demux2/3 -> Relational Operator/1, Relational Operator1/1
  Demux2/2 -> Relational Operator/2
  Demux2/1 -> Relational Operator1/2
  Data Type Conversion/1 -> C/1

== system wt_blockset_v3/Power Converters/3-phase Diode Bridge Rectifier/Diode  State Calculator/Branch C- ==
  RST : Inport  Port=1  LatchInput=off
  Data Type Conversion : DataTypeConversion
  Demux2 : Demux  Outputs=3
  Logical Operator : Logic
  Relational Operator : RelationalOperator  Operator=<  InputSameDT=on
  Relational Operator1 : RelationalOperator  Operator=<  InputSameDT=on
  C : Outport  InitialOutput=0
  wires:
  Demux2/1 -> Relational Operator1/2
  Demux2/2 -> Relational Operator/2
  Demux2/3 -> Relational Operator1/1, Relational Operator/1
  RST/1 -> Demux2/1
  Logical Operator/1 -> Data Type Conversion/1
  Relational Operator1/1 -> Logical Operator/2
  Relational Operator/1 -> Logical Operator/1
  Data Type Conversion/1 -> C/1

== system wt_blockset_v3/Power Converters/Average SVM Strategy/1st quadrant/Sector 0 ==
  note: Sector 0
  vd : Inport  Port=1  LatchInput=off
  vq : Inport  Port=2  LatchInput=off
  Action Port : ActionPort  InitializeStates=reset
  Constant : Constant  Value=0.5
  Mux : Mux  Inputs=3
  Mux1 : Mux  Inputs=3
  Mux2 : Mux  Inputs=3
  Mux3 : Mux  Inputs=2
  Sum : Sum  Inputs=-+-  SaturateOnIntegerOverflow=on
  T0_pr : Fcn  Expr=(u(2)<=0)*0+(u(2)>0)*u(2)
  T1_pr : Fcn  Expr=(u(2)<=0)*(0.5*u(1)/(u(1)+u(3)))+(u(2)>0)*u(1)
  T2_pr : Fcn  Expr=(u(2)<=0)*(0.5*u(3)/(u(1)+u(3)))+(u(2)>0)*u(3)
  T_1 : Fcn  Expr=0.5*(u(1)-u(2)/sqrt(3))
  T_2 : Fcn  Expr=u(2)/sqrt(3)
  duty_A : Fcn  Expr=1-u(3)
  duty_B : Fcn  Expr=1-(u(3)+2*u(1))
  duty_C : Fcn  Expr=u(3)
  duty_ABC : Outport  OutputWhenDisabled=reset  InitialOutput=[0 0 0]
  wires:
  T_2/1 -> Sum/3, Mux1/3
  T_1/1 -> Sum/1, Mux1/1
  Constant/1 -> Sum/2
  Sum/1 -> Mux1/2
  T1_pr/1 -> [T1]
  T2_pr/1 -> [T2]
  T0_pr/1 -> [T0]
  Mux1/1 -> T1_pr/1, T2_pr/1, T0_pr/1
  [T1] -> Mux2/1
  [T2] -> Mux2/2
  [T0] -> Mux2/3
  Mux2/1 -> duty_B/1, duty_A/1, duty_C/1
  duty_A/1 -> Mux/1
  duty_B/1 -> Mux/2
  duty_C/1 -> Mux/3
  Mux/1 -> duty_ABC/1
  Mux3/1 -> T_1/1, T_2/1
  vd/1 -> Mux3/1
  vq/1 -> Mux3/2

== system wt_blockset_v3/Power Converters/Average SVM Strategy/1st quadrant/Sector 1 ==
  note: Sector 1
  vd : Inport  Port=1  LatchInput=off
  vq : Inport  Port=2  LatchInput=off
  Action Port : ActionPort  InitializeStates=reset
  Constant : Constant  Value=0.5
  Mux : Mux  Inputs=3
  Mux1 : Mux  Inputs=3
  Mux2 : Mux  Inputs=3
  Mux3 : Mux  Inputs=2
  Sum : Sum  Inputs=-+-  SaturateOnIntegerOverflow=on
  T0_pr : Fcn  Expr=(u(2)<=0)*0+(u(2)>0)*u(2)
  T1_pr : Fcn  Expr=(u(2)<=0)*(0.5*u(1)/(u(1)+u(3)))+(u(2)>0)*u(1)
  T2_pr : Fcn  Expr=(u(2)<=0)*(0.5*u(3)/(u(1)+u(3)))+(u(2)>0)*u(3)
  T_1 : Fcn  Expr=0.5*(-u(1)+u(2)/sqrt(3))
  T_2 : Fcn  Expr=0.5*(+u(1)+u(2)/sqrt(3))
  duty_A : Fcn  Expr=1-(u(3)+2*u(1))
  duty_B : Fcn  Expr=1-u(3)
  duty_C : Fcn  Expr=u(3)
  duty_ABC : Outport  OutputWhenDisabled=reset  InitialOutput=[0 0 0]
  wires:
  Sum/1 -> Mux1/2
  Constant/1 -> Sum/2
  T_1/1 -> Sum/1, Mux1/1
  T_2/1 -> Mux1/3, Sum/3
  Mux1/1 -> T1_pr/1, T2_pr/1, T0_pr/1
  T1_pr/1 -> [T1]
  T2_pr/1 -> [T2]
  T0_pr/1 -> [T0]
  [T1] -> Mux2/1
  [T2] -> Mux2/2
  [T0] -> Mux2/3
  Mux/1 -> duty_ABC/1
  Mux2/1 -> duty_B/1, duty_A/1, duty_C/1
  duty_B/1 -> Mux/2
  duty_A/1 -> Mux/1
  duty_C/1 -> Mux/3
  Mux3/1 -> T_1/1, T_2/1
  vq/1 -> Mux3/2
  vd/1 -> Mux3/1

== system wt_blockset_v3/Power Converters/Average SVM Strategy/2nd quadrant/Sector 1 ==
  note: Sector 1
  vd : Inport  Port=1  LatchInput=off
  vq : Inport  Port=2  LatchInput=off
  Action Port : ActionPort  InitializeStates=reset
  Constant : Constant  Value=0.5
  Mux : Mux  Inputs=3
  Mux1 : Mux  Inputs=3
  Mux2 : Mux  Inputs=3
  Mux3 : Mux  Inputs=2
  Sum : Sum  Inputs=-+-  SaturateOnIntegerOverflow=on
  T0_pr : Fcn  Expr=(u(2)<=0)*0+(u(2)>0)*u(2)
  T1_pr : Fcn  Expr=(u(2)<=0)*(0.5*u(1)/(u(1)+u(3)))+(u(2)>0)*u(1)
  T2_pr : Fcn  Expr=(u(2)<=0)*(0.5*u(3)/(u(1)+u(3)))+(u(2)>0)*u(3)
  T_1 : Fcn  Expr=0.5*(-u(1)+u(2)/sqrt(3))
  T_2 : Fcn  Expr=0.5*(+u(1)+u(2)/sqrt(3))
  duty_A : Fcn  Expr=1-(u(3)+2*u(1))
  duty_B : Fcn  Expr=1-u(3)
  duty_C : Fcn  Expr=u(3)
  duty_ABC : Outport  OutputWhenDisabled=reset  InitialOutput=[0 0 0]
  wires:
  Sum/1 -> Mux1/2
  Constant/1 -> Sum/2
  T_1/1 -> Sum/1, Mux1/1
  T_2/1 -> Mux1/3, Sum/3
  Mux1/1 -> T1_pr/1, T2_pr/1, T0_pr/1
  T1_pr/1 -> [T1]
  T2_pr/1 -> [T2]
  T0_pr/1 -> [T0]
  [T1] -> Mux2/1
  [T2] -> Mux2/2
  [T0] -> Mux2/3
  Mux/1 -> duty_ABC/1
  Mux2/1 -> duty_B/1, duty_A/1, duty_C/1
  duty_B/1 -> Mux/2
  duty_A/1 -> Mux/1
  duty_C/1 -> Mux/3
  Mux3/1 -> T_1/1, T_2/1
  vq/1 -> Mux3/2
  vd/1 -> Mux3/1

== system wt_blockset_v3/Power Converters/Average SVM Strategy/2nd quadrant/Sector 2 ==
  note: Sector 2
  vd : Inport  Port=1  LatchInput=off
  vq : Inport  Port=2  LatchInput=off
  Action Port : ActionPort  InitializeStates=reset
  Constant : Constant  Value=0.5
  Mux : Mux  Inputs=3
  Mux1 : Mux  Inputs=3
  Mux2 : Mux  Inputs=3
  Mux3 : Mux  Inputs=2
  Sum : Sum  Inputs=-+-  SaturateOnIntegerOverflow=on
  T0_pr : Fcn  Expr=(u(2)<=0)*0+(u(2)>0)*u(2)
  T1_pr : Fcn  Expr=(u(2)<=0)*(0.5*u(1)/(u(1)+u(3)))+(u(2)>0)*u(1)
  T2_pr : Fcn  Expr=(u(2)<=0)*(0.5*u(3)/(u(1)+u(3)))+(u(2)>0)*u(3)
  T_ : Fcn  Expr=0.5*(abs(u(1))-u(2)/sqrt(3))
  T_1 : Fcn  Expr=u(2)/sqrt(3)
  duty_A : Fcn  Expr=u(3)
  duty_B : Fcn  Expr=1-u(3)
  duty_C : Fcn  Expr=1-(u(3)+2*u(1))
  duty_ABC : Outport  OutputWhenDisabled=reset  InitialOutput=[0 0 0]
  wires:
  Mux/1 -> duty_ABC/1
  [T0] -> Mux2/3
  [T2] -> Mux2/2
  [T1] -> Mux2/1
  Mux1/1 -> T0_pr/1, T2_pr/1, T1_pr/1
  T0_pr/1 -> [T0]
  T2_pr/1 -> [T2]
  T1_pr/1 -> [T1]
  Sum/1 -> Mux1/2
  Constant/1 -> Sum/2
  vq/1 -> Mux3/2
  vd/1 -> Mux3/1
  Mux3/1 -> T_1/1, T_/1
  T_1/1 -> Mux1/1, Sum/1
  T_/1 -> Mux1/3, Sum/3
  duty_B/1 -> Mux/2
  duty_A/1 -> Mux/1
  duty_C/1 -> Mux/3
  Mux2/1 -> duty_B/1, duty_A/1, duty_C/1

== system wt_blockset_v3/Power Converters/Average SVM Strategy/3rd quadrant/Sector 3 ==
  note: Sector 2
  vd : Inport  Port=1  LatchInput=off
  vq : Inport  Port=2  LatchInput=off
  Action Port : ActionPort  InitializeStates=reset
  Constant : Constant  Value=0.5
  Mux : Mux  Inputs=3
  Mux1 : Mux  Inputs=3
  Mux2 : Mux  Inputs=3
  Mux3 : Mux  Inputs=2
  Sum : Sum  Inputs=-+-  SaturateOnIntegerOverflow=on
  T0_pr : Fcn  Expr=(u(2)<=0)*0+(u(2)>0)*u(2)
  T1_pr : Fcn  Expr=(u(2)<=0)*(0.5*u(1)/(u(1)+u(3)))+(u(2)>0)*u(1)
  T2_pr : Fcn  Expr=(u(2)<=0)*(0.5*u(3)/(u(1)+u(3)))+(u(2)>0)*u(3)
  T_ : Fcn  Expr=0.5*(abs(u(1))-abs(u(2))/sqrt(3))
  T_1 : Fcn  Expr=abs(u(2))/sqrt(3)
  duty_A : Fcn  Expr=u(3)
  duty_B : Fcn  Expr=1-(u(3)+2*u(1))
  duty_C : Fcn  Expr=1-u(3)
  duty_ABC : Outport  OutputWhenDisabled=reset  InitialOutput=[0 0 0]
  wires:
  Mux/1 -> duty_ABC/1
  [T0] -> Mux2/3
  [T2] -> Mux2/2
  [T1] -> Mux2/1
  Mux1/1 -> T0_pr/1, T2_pr/1, T1_pr/1
  T0_pr/1 -> [T0]
  T2_pr/1 -> [T2]
  T1_pr/1 -> [T1]
  Sum/1 -> Mux1/2
  Constant/1 -> Sum/2
  vq/1 -> Mux3/2
  vd/1 -> Mux3/1
  Mux3/1 -> T_1/1, T_/1
  T_1/1 -> Mux1/1, Sum/1
  T_/1 -> Mux1/3, Sum/3
  duty_A/1 -> Mux/1
  Mux2/1 -> duty_A/1, duty_B/1, duty_C/1
  duty_B/1 -> Mux/2
  duty_C/1 -> Mux/3
